simulink model "motorsPID"  (R2015a)
settings: Solver=ode45  StartTime=0.0  StopTime=Tsim  RelTol=1e-3
values from neighbouring files (symbols this model uses):
  b = m*(2.0*pi/L)    [GenPath.m]    (also in simula_robo.m = 0.1)
  d = 0.4    [simula_robo.m]
  J = 0.01    [simula_robo.m]
  Kd = 0    [simula_robo.m]
  Ke = 0.08    [simula_robo.m]
  Ki = 10.0    (= 10)    [simula_robo.m]
  Kp = 5.0    (= 5)    [simula_robo.m]
  L = input('Entre o comprimento máximo: ')    [GenPath.m]    (also in Nepsac_DeltaU.m = L(1:2*Nu,:); simula_robo.m = 0.5)
  R = 0.01*eye(2*Nu)    [Nepsac_DeltaU.m]    (also in simula_robo.m = 1)
  thetao = 0    [simula_robo.m]
  Ts = 0.1    [GenPath.m]    (also in modelo.m; simula_robo.m)
  xo = p    [GenPath.m]    (also in Nepsac_DeltaU.m = [u(7);u(8);u(9)]; modelo.m = x; simula_robo.m = 0)
  yo = 0    [simula_robo.m]
libraries: simulink_extras x2, simulink x2
settings Model: Creator=Thiago  LastModifiedBy=Thiago

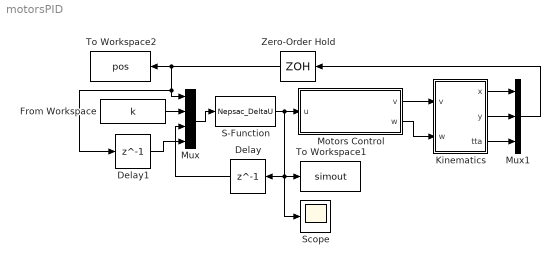
== system motorsPID ==
  Delay : Delay  DelayLength=1  SampleTime=Ts
  Delay1 : Delay  DelayLength=1  SampleTime=Ts
  From Workspace : FromWorkspace  VariableName=k  SampleTime=0.1
  Kinematics : Subsystem
  Motors Control : Subsystem
  Mux : Mux
  Mux1 : Mux  Inputs=3
  S-Function : S-Function  FunctionName=Nepsac_DeltaU
  Scope : Scope
  To Workspace1 : ToWorkspace  VariableName=simout  SaveFormat=Structure With Time  SampleTime=-1
  To Workspace2 : ToWorkspace  VariableName=pos  SaveFormat=Structure With Time  SampleTime=-1
  Zero-Order Hold : ZeroOrderHold  SampleTime=0.1
  wires:
  S-Function/1 -> Scope/1, To Workspace1/1, Delay/1, Motors Control/1(u)
  Motors Control/1(v) -> Kinematics/1(v)
  Motors Control/2(w) -> Kinematics/2(w)
  Kinematics/1(x) -> Mux1/1
  Kinematics/2(y) -> Mux1/2
  Kinematics/3(tta) -> Mux1/3
  Mux/1 -> S-Function/1
  Mux1/1 -> Zero-Order Hold/1
  From Workspace/1 -> Mux/2
  Delay/1 -> Mux/3
  Delay1/1 -> Mux/4
  Zero-Order Hold/1 -> To Workspace2/1, Delay1/1, Mux/1

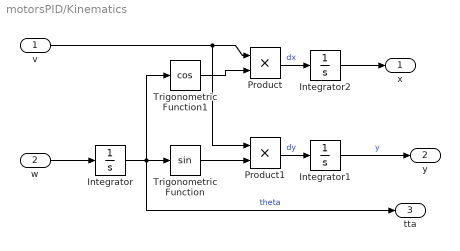
== system motorsPID/Kinematics ==
  v : Inport
  w : Inport  Port=2
  Integrator : Integrator  InitialCondition=thetao
  Integrator1 : Integrator  InitialCondition=yo
  Integrator2 : Integrator  InitialCondition=xo
  Product : Product
  Product1 : Product
  Trigonometric Function : Trigonometry
  Trigonometric Function1 : Trigonometry  Operator=cos
  x : Outport
  y : Outport  Port=2
  tta : Outport  Port=3
  wires:
  v/1 -> Product1/1, Product/1
  Trigonometric Function1/1 -> Product/2
  Product/1 -> Integrator2/1  "dx"
  Integrator/1 -> tta/1, Trigonometric Function1/1, Trigonometric Function/1  "theta"
  Integrator1/1 -> y/1  "y"
  Product1/1 -> Integrator1/1  "dy"
  Trigonometric Function/1 -> Product1/2
  Integrator2/1 -> x/1
  w/1 -> Integrator/1

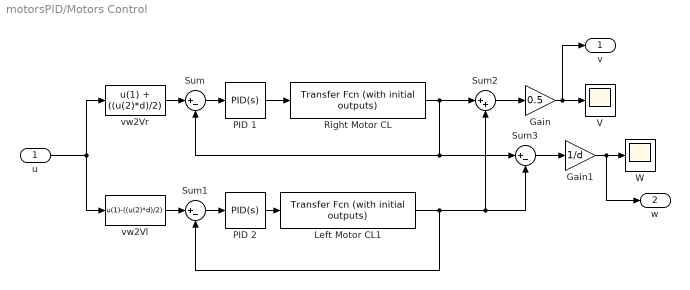
== system motorsPID/Motors Control ==
  u : Inport
  Gain : Gain  Gain=0.5
  Gain1 : Gain  Gain=1/d
  Left Motor CL1 : simulink_extras/Additional Linear/Transfer Fcn (with initial outputs)  N=[Ke]  D="[J*L  (J*R+b*L) (b*R+Ke^2)]"  Y0=0  U0=0
  PID 1 : simulink/Continuous/PID Controller  Controller=PID  TimeDomain=Continuous-time  SampleTime=-1  IntegratorMethod=Forward Euler  FilterMethod=Forward Euler  Form=Parallel  UseFilter=on  ControllerParametersSource=internal  P=Kp  I=Ki  D=Kd  N=100  InitialConditionSource=internal  InitialConditionForIntegrator=0  InitialConditionForFilter=0  ExternalReset=none  LimitOutput=off  UpperSaturationLimit=inf  LowerSaturationLimit=-inf  LinearizeAsGain=on  AntiWindupMode=none  Kb=1  TrackingMode=off  Kt=1  PParamMin=[]  PParamMax=[]  IParamMin=[]  IParamMax=[]  DParamMin=[]  DParamMax=[]  NParamMin=[]  NParamMax=[]  KbParamMin=[]  KbParamMax=[]  KtParamMin=[]  KtParamMax=[]  POutMin=[]  POutMax=[]  IOutMin=[]  IOutMax=[]  DOutMin=[]  DOutMax=[]  NOutMin=[]  NOutMax=[]  KbOutMin=[]  KbOutMax=[]  KtOutMin=[]  KtOutMax=[]  IntegratorOutMin=[]  IntegratorOutMax=[]  FilterOutMin=[]  FilterOutMax=[]  SumOutMin=[]  SumOutMax=[]  SumI1OutMin=[]  SumI1OutMax=[]  SumI2OutMin=[]  SumI2OutMax=[]  SumI3OutMin=[]  SumI3OutMax=[]  SumDOutMin=[]  SumDOutMax=[]  SaturationOutMin=[]  SaturationOutMax=[]  IntegratorContinuousStateAttributes=''  IntegratorStateMustResolveToSignalObject=off  IntegratorRTWStateStorageClass=Auto  FilterContinuousStateAttributes=''  FilterStateMustResolveToSignalObject=off  FilterRTWStateStorageClass=Auto  DifferentiatorICPrevScaledInput=0  DifferentiatorOutMin=[]  DifferentiatorOutMax=[]
  PID 2 : simulink/Continuous/PID Controller  Controller=PID  TimeDomain=Continuous-time  SampleTime=-1  IntegratorMethod=Forward Euler  FilterMethod=Forward Euler  Form=Parallel  UseFilter=on  ControllerParametersSource=internal  P=Kp  I=Ki  D=Kd  N=100  InitialConditionSource=internal  InitialConditionForIntegrator=0  InitialConditionForFilter=0  ExternalReset=none  LimitOutput=off  UpperSaturationLimit=inf  LowerSaturationLimit=-inf  LinearizeAsGain=on  AntiWindupMode=none  Kb=1  TrackingMode=off  Kt=1  PParamMin=[]  PParamMax=[]  IParamMin=[]  IParamMax=[]  DParamMin=[]  DParamMax=[]  NParamMin=[]  NParamMax=[]  KbParamMin=[]  KbParamMax=[]  KtParamMin=[]  KtParamMax=[]  POutMin=[]  POutMax=[]  IOutMin=[]  IOutMax=[]  DOutMin=[]  DOutMax=[]  NOutMin=[]  NOutMax=[]  KbOutMin=[]  KbOutMax=[]  KtOutMin=[]  KtOutMax=[]  IntegratorOutMin=[]  IntegratorOutMax=[]  FilterOutMin=[]  FilterOutMax=[]  SumOutMin=[]  SumOutMax=[]  SumI1OutMin=[]  SumI1OutMax=[]  SumI2OutMin=[]  SumI2OutMax=[]  SumI3OutMin=[]  SumI3OutMax=[]  SumDOutMin=[]  SumDOutMax=[]  SaturationOutMin=[]  SaturationOutMax=[]  IntegratorContinuousStateAttributes=''  IntegratorStateMustResolveToSignalObject=off  IntegratorRTWStateStorageClass=Auto  FilterContinuousStateAttributes=''  FilterStateMustResolveToSignalObject=off  FilterRTWStateStorageClass=Auto  DifferentiatorICPrevScaledInput=0  DifferentiatorOutMin=[]  DifferentiatorOutMax=[]
  Right Motor CL : simulink_extras/Additional Linear/Transfer Fcn (with initial outputs)  N=[Ke]  D="[J*L  (J*R+b*L) (b*R+Ke^2)]"  Y0=0  U0=0
  Sum : Sum  Inputs=|+-
  Sum1 : Sum  Inputs=|+-
  Sum2 : Sum  Inputs=|++
  Sum3 : Sum  Inputs=|+-
  V : Scope
  W : Scope
      settings: SaveName=ScopeData2
  vw2Vl : Fcn  Expr=u(1)-((u(2)*d)/2)
  vw2Vr : Fcn  Expr=u(1) + ((u(2)*d)/2)
  v : Outport
  w : Outport  Port=2
  wires:
  u/1 -> vw2Vr/1, vw2Vl/1
  PID 1/1 -> Right Motor CL/1
  Sum/1 -> PID 1/1
  PID 2/1 -> Left Motor CL1/1
  Sum1/1 -> PID 2/1
  vw2Vl/1 -> Sum1/1
  Left Motor CL1/1 -> Sum3/2, Sum2/2, Sum1/2
  vw2Vr/1 -> Sum/1
  Right Motor CL/1 -> Sum2/1, Sum3/1, Sum/2
  Gain/1 -> v/1, V/1
  Sum2/1 -> Gain/1
  Sum3/1 -> Gain1/1
  Gain1/1 -> w/1, W/1
